simulink model "Testbench_for_Power_Circulating_TopologyA"  (R2023b)
settings: Solver=VariableStepAuto  StartTime=0.0  StopTime=4  RelTol=1e-3
InitFcn:
  | Initialization_for_Testbench;
values from neighbouring files (symbols this model uses):
  Cdc = 180e-6    (= 0.00018)    [CurrentLoop.m]    (also in Initialization_for_ESS_3P_2L_220kW.m; Initialization_for_Testbench.m)
  Fnom_Grid = 50    [CurrentLoop.m]    (also in Initialization_for_ESS_3P_2L_220kW.m; Initialization_for_Testbench.m)
  Gain_for_ActiveDamping = 1    [Initialization_for_Testbench.m]
  Inom = Pnom/sqrt(3)/Unom_Grid    [CurrentLoop.m]    (also in Initialization_for_ESS_3P_2L_220kW.m; Initialization_for_Testbench.m)
  Ki_Idq = Kp_Idq*2*pi*2    (= 40.2123859659)    [Initialization_for_ESS_3P_2L_220kW.m]    (also in Initialization_for_Testbench.m = 1.26330936334)
  Ki_Udc = Kp_Udc*2*pi*10    (= 6283.18530718)    [Initialization_for_Testbench.m]
  Kp_Idq = L_grid/3/Ts_Control*3    (= 3.2)    [Initialization_for_ESS_3P_2L_220kW.m]    (also in Initialization_for_Testbench.m = 2.0106192983)
  Kp_Udc = 100    [Initialization_for_Testbench.m]
  L_grid = 200e-6    (= 0.0002)    [Initialization_for_ESS_3P_2L_220kW.m]    (also in Initialization_for_Testbench.m)
  Pnom = 220e3    (= 220000)    [CurrentLoop.m]    (also in Initialization_for_ESS_3P_2L_220kW.m; Initialization_for_Testbench.m = 2500000)
  Ts_Control = 62.5e-6    (= 6.25e-05)    [CurrentLoop.m]    (also in Initialization_for_ESS_3P_2L_220kW.m; Initialization_for_Testbench.m = 0.0001)
  Ts_Power = 10e-7    (= 1e-06)    [Initialization_for_ESS_3P_2L_220kW.m]    (also in Initialization_for_Testbench.m)
  Udc_ref = 1500    [CurrentLoop.m]    (also in Initialization_for_ESS_3P_2L_220kW.m; Initialization_for_Testbench.m)
  Unom_Grid = 690    [CurrentLoop.m]    (also in Initialization_for_ESS_3P_2L_220kW.m; Initialization_for_Testbench.m)
  Unom_Phase = Unom_Grid/sqrt(3)    [CurrentLoop.m]    (also in Initialization_for_ESS_3P_2L_220kW.m; Initialization_for_Testbench.m)
libraries: LibraryForCodeGeneration x35, spsSeriesRLCBranchLib x3, spsThreePhaseVIMeasurementLib x3, spsTriangleGeneratorLib x2, spsThreePhaseSeriesRLCBranchLib x2, spsUniversalBridgeLib x2, eeProgrammableSignalGenerator x1, spsStairGeneratorLib x1, spsThreePhaseSourceLib x1, spsVoltageMeasurementLib x1, spspowerguiLib x1
settings Model: DataDictionary=VariablesDictionary_for_Testbench_TopologyA.sldd  Creator=ZZY  LastModifiedBy=ZZY

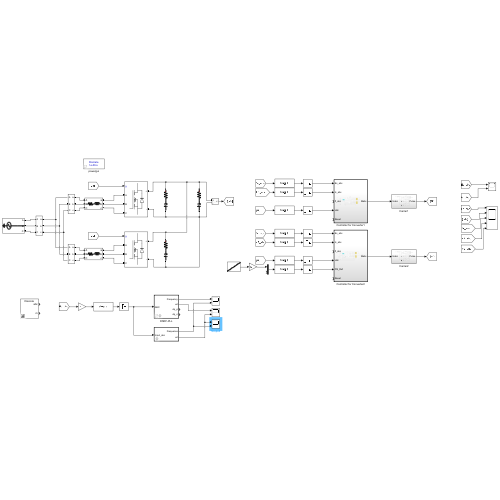
[thumbnail: Simulink's stored preview of the top-level diagram]
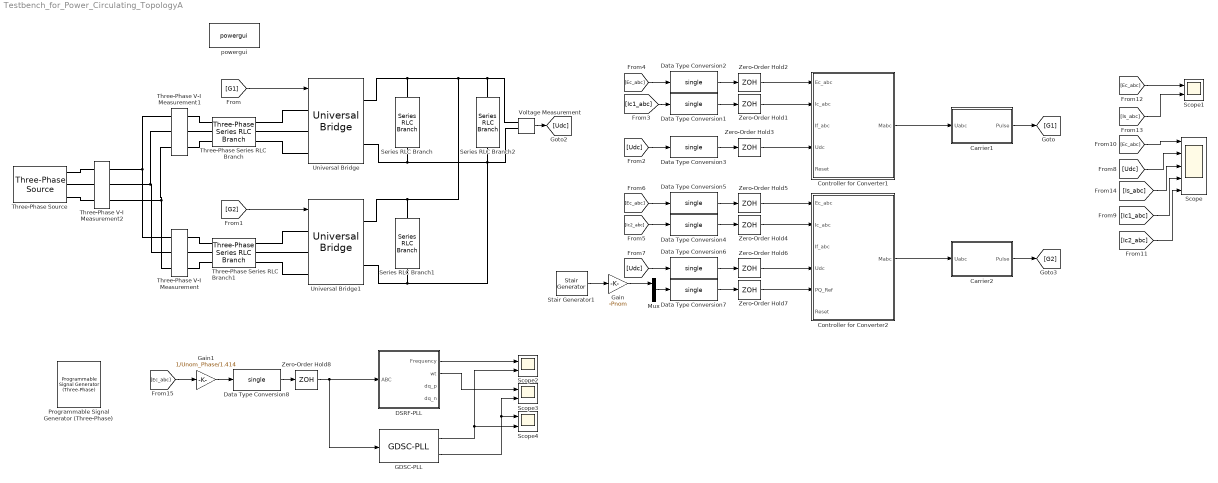
== system Testbench_for_Power_Circulating_TopologyA ==
  Carrier1 : Subsystem
  Carrier2 : Subsystem
  Controller for Converter1 : Subsystem  TreatAsAtomicUnit=on  SystemSampleTime=Ts_Control
  Controller for Converter2 : Subsystem  TreatAsAtomicUnit=on  SystemSampleTime=Ts_Control
  DSRF-PLL : Subsystem  AncestorBlock=LibraryForCodeGeneration/DSRF-PLL  TreatAsAtomicUnit=on  RTWFcnName=DSRF_PLL  mask{Ts=Ts_Control}
      mask prompts: Ts "Sampling Time:"
      settings: RTWFcnNameOpts=User specified
  Data Type Conversion{1..8} (8 alike) : DataTypeConversion  OutDataTypeStr=single  SaturateOnIntegerOverflow=off  RndMeth=Floor
  GDSC-PLL : LibraryForCodeGeneration/GDSC-PLL  Ts=Ts_Control  Fnom_Grid=50
  Gain : Gain  Gain=-Pnom
  Gain1 : Gain  Gain=1/Unom_Phase/1.414
  Mux : Mux  Inputs=2
  Programmable Signal Generator (Three-Phase) : eeProgrammableSignalGenerator/Programmable Signal Generator (Three-Phase)  LabelModeActiveChoice=Discrete  VariationAmplitude=Constant  Amp=0.8  Amp_RampRate=100  Amp_StepValue=100  Amp_ModulationMag=50  Amp_ModulationFreq=10  Amp_Tstart=0.1  Amp_Tstop=0.6  Amp_Table=[0 30 60 90]  Amp_Time=[0 0.3 0.6 0.9]  VariationFrequency=Constant  Freq=50  Freq_RampRate=100  Freq_StepValue=100  Freq_ModulationMag=50  Freq_ModulationFreq=10  Freq_Tstart=0.1  Freq_Tstop=0.6  Freq_Table=[0 30 60 90]  Freq_Time=[0 0.3 0.6 0.9]  VariationPhase=Constant  Phase=0  Phase_RampRate=100  Phase_StepValue=100  Phase_ModulationMag=50  Phase_ModulationFreq=10  Phase_Tstart=0.1  Phase_Tstop=0.6  Phase_Table=[0 30 60 90]  Phase_Time=[0 0.3 0.6 0.9]  Harmo_En1=on  Harmo_Seq1=Negative Sequence  Harmo_Ord1=2  Harmo_Mag1=0.4  Harmo_Phase1=180  Harmo_Tstart1=0.1  Harmo_Tstop1=0.6  Harmo_En2=on  Harmo_Seq2=Negative Sequence  Harmo_Ord2=3  Harmo_Mag2=0.4  Harmo_Phase2=180  Harmo_Tstart2=0.3  Harmo_Tstop2=1  Ts=Ts_Control
      settings: LibrarySourceBlock=|
      | ee_sl_lib/General Control/Programmable
      | Signal Generator (Three-Phase)
  Scope : Scope  NumInputPorts=5
  Scope{1..4} (4 alike) : Scope  NumInputPorts=2
  Series RLC Branch : spsSeriesRLCBranchLib/Series RLC Branch  LConnTagsString=__new0  RConnTagsString=__new0  BranchType=RC  Resistance=1e-6  Inductance=1e-3  SetiL0=off  InitialCurrent=0  Capacitance=Cdc  Setx0=on  InitialVoltage=Udc_ref  Measurements=Branch voltage
  Series RLC Branch1 : spsSeriesRLCBranchLib/Series RLC Branch  LConnTagsString=__new0  RConnTagsString=__new0  BranchType=RC  Resistance=1e-6  Inductance=1e-3  SetiL0=off  InitialCurrent=0  Capacitance=Cdc  Setx0=on  InitialVoltage=Udc_ref  Measurements=Branch voltage
  Series RLC Branch2 : spsSeriesRLCBranchLib/Series RLC Branch  LConnTagsString=__new0  RConnTagsString=__new0  BranchType=RC  Resistance=1e-6  Inductance=1e-3  SetiL0=off  InitialCurrent=0  Capacitance=Cdc*1000  Setx0=on  InitialVoltage=Udc_ref  Measurements=Branch voltage
  Stair Generator1 : spsStairGeneratorLib/Stair Generator  t=0:0.2:2  e=0:0.1:1  Ts=0
  Three-Phase Series RLC Branch : spsThreePhaseSeriesRLCBranchLib/Three-Phase Series RLC Branch  LConnTagsString=A|B|C  RConnTagsString=A|B|C  BranchType=RL  Resistance=1e-3  Inductance=L_grid*1  Capacitance=1e-6  Measurements=None
  Three-Phase Series RLC Branch1 : spsThreePhaseSeriesRLCBranchLib/Three-Phase Series RLC Branch  LConnTagsString=A|B|C  RConnTagsString=A|B|C  BranchType=RL  Resistance=1e-3  Inductance=L_grid*1  Capacitance=1e-6  Measurements=None
  Three-Phase V-I Measurement : spsThreePhaseVIMeasurementLib/Three-Phase V-I Measurement  VoltageMeasurement=no  SetLabelV=off  LabelV=Vabc  Vpu=off  VpuLL=off  CurrentMeasurement=yes  SetLabelI=on  LabelI=Ic2_abc  Ipu=off  Pbase=100e6  Vbase=500e3  OutputType=Complex  PhasorSimulation=off  PSBequivalent=0
  Three-Phase V-I Measurement1 : spsThreePhaseVIMeasurementLib/Three-Phase V-I Measurement  VoltageMeasurement=phase-to-phase  SetLabelV=on  LabelV=Ec_abc  Vpu=off  VpuLL=off  CurrentMeasurement=yes  SetLabelI=on  LabelI=Ic1_abc  Ipu=off  Pbase=100e6  Vbase=500e3  OutputType=Complex  PhasorSimulation=off  PSBequivalent=0
  Three-Phase V-I Measurement2 : spsThreePhaseVIMeasurementLib/Three-Phase V-I Measurement  VoltageMeasurement=no  SetLabelV=off  LabelV=Ec_abc  Vpu=off  VpuLL=off  CurrentMeasurement=yes  SetLabelI=on  LabelI=Is_abc  Ipu=off  Pbase=100e6  Vbase=500e3  OutputType=Complex  PhasorSimulation=off  PSBequivalent=0
  Three-Phase Source : spsThreePhaseSourceLib/Three-Phase Source  InternalConnection=Yg  VoltagePhases=off  Voltage=Unom_Grid  PhaseAngle=0  Voltage_phases=[25e3 25e3 25e3]/sqrt(3)  PhaseAngles_phases=[0 -120 +120]  Frequency=50  NonIdealSource=off  SpecifyImpedance=off  Resistance=0.08929  Inductance=2e-3  ShortCircuitLevel=100e6  BaseVoltage=Unom_Grid  XRratio=7  BusType=swing  Pref=10e3  Qref=0  Prefabc=[10e3, 10e3, 10e3]  Qrefabc=[0, 0, 0]  Qmin=-inf  Qmax=inf
  Universal Bridge : spsUniversalBridgeLib/Universal Bridge  Arms=3  SnubberResistance=1e5  SnubberCapacitance=inf  Device=MOSFET / Diodes  Ron=1e-3  Lon=0  ForwardVoltages="[  0  0  ]"  ForwardVoltage=0  GTOparameters=[ 10e-6 , 20e-6 ]  IGBTparameters=[ 1e-6 , 2e-6 ]  Measurements=None  Measurements_2=None  converterType=Rectifier
  Universal Bridge1 : spsUniversalBridgeLib/Universal Bridge  Arms=3  SnubberResistance=1e5  SnubberCapacitance=inf  Device=MOSFET / Diodes  Ron=1e-3  Lon=0  ForwardVoltages="[  0  0  ]"  ForwardVoltage=0  GTOparameters=[ 10e-6 , 20e-6 ]  IGBTparameters=[ 1e-6 , 2e-6 ]  Measurements=None  Measurements_2=None  converterType=Rectifier
  Voltage Measurement : spsVoltageMeasurementLib/Voltage Measurement  PhasorSimulation=off  OutputType=Complex  PSBequivalent=0
  Zero-Order Hold{1..8} (8 alike) : ZeroOrderHold  SampleTime=Ts_Control
  powergui : spspowerguiLib/powergui  Priority=1  SimulationMode=Discrete  SampleTime=Ts_Power  frequency=60  Iterations=50  frequencyindice=0  Pbase=100e6  ErrMax=1e-4  UnitsV=kV  UnitsW=MW  buscounter=0  FunctionMessages=off  echomessages=off  EnableUseOfTLC=off  CurrentSourceSwitches=off  DisableSnubberDevices=off  DisableRonSwitches=off  DisableVfSwitches=off  DisplayEquations=off  AutomaticDiscreteSolvers=off  SolverType=Tustin/Backward Euler (TBE)  Interpol=off  ExternalGateDelay=off  methode=off  Ts=100  x0status=blocks  SPID=on  SwTol=0  HookPort=off  NonlinearTolerance=1e-4  nMaxIteration=100  ContinueOnMaxIteration=off  RestoreLinks=warning  ResistiveCurrentMeasurement=off  Frange=[0:2:500]  Ylog=off  Xlog=on  ShowGrid=off  save=off  variable=ZData  structure=CHB_abc  ZoomFFT=off  StartTime=1.4  cycles=5  DisplayStyle=1  fundamental=50  FreqAxis=off  MaxFrequency=30000  frequencyindicesteady=1  RmsSteady=1  display=off
  wires:
  [G1] -> Universal Bridge/1
  [G2] -> Universal Bridge1/1
  Voltage Measurement/1 -> [Udc]
  Carrier1/1(Pulse) -> [G1]
  Carrier2/1(Pulse) -> [G2]
  Controller for Converter1/1(Mabc) -> Carrier1/1(Uabc)
  Controller for Converter2/1(Mabc) -> Carrier2/1(Uabc)
  Data Type Conversion3/1 -> Zero-Order Hold3/1
  [Udc] -> Data Type Conversion3/1
  Zero-Order Hold3/1 -> Controller for Converter1/4(Udc)
  [Ic1_abc] -> Data Type Conversion1/1
  Data Type Conversion1/1 -> Zero-Order Hold1/1
  Data Type Conversion2/1 -> Zero-Order Hold2/1
  [Ec_abc] -> Data Type Conversion2/1
  Zero-Order Hold2/1 -> Controller for Converter1/1(Ec_abc)
  Zero-Order Hold1/1 -> Controller for Converter1/2(Ic_abc)
  Data Type Conversion5/1 -> Zero-Order Hold5/1
  [Ic2_abc] -> Data Type Conversion4/1
  Data Type Conversion4/1 -> Zero-Order Hold4/1
  [Ec_abc] -> Data Type Conversion5/1
  Zero-Order Hold5/1 -> Controller for Converter2/1(Ec_abc)
  Zero-Order Hold4/1 -> Controller for Converter2/2(Ic_abc)
  Data Type Conversion6/1 -> Zero-Order Hold6/1
  [Udc] -> Data Type Conversion6/1
  Zero-Order Hold6/1 -> Controller for Converter2/4(Udc)
  [Udc] -> Scope/2
  [Ic1_abc] -> Scope/4
  [Ec_abc] -> Scope/1
  [Ic2_abc] -> Scope/5
  Mux/1 -> Data Type Conversion7/1
  Data Type Conversion7/1 -> Zero-Order Hold7/1
  Zero-Order Hold7/1 -> Controller for Converter2/5(PQ_Ref)
  Gain/1 -> Mux/1
  Stair Generator1/1 -> Gain/1
  [Ec_abc] -> Scope1/1
  [Is_abc] -> Scope1/2
  [Is_abc] -> Scope/3
  [Ec_abc] -> Gain1/1
  Data Type Conversion8/1 -> Zero-Order Hold8/1
  DSRF-PLL/1(Frequency) -> Scope2/1
  GDSC-PLL/1 -> Scope4/2, Scope2/2
  DSRF-PLL/2(wt) -> Scope3/1
  GDSC-PLL/2 -> Scope4/1, Scope3/2
  Zero-Order Hold8/1 -> GDSC-PLL/1, DSRF-PLL/1(ABC)
  Gain1/1 -> Data Type Conversion8/1
  connections:
  Series RLC Branch1/LConn1 -- Series RLC Branch2/LConn1 -- Voltage Measurement/LConn1 -- Universal Bridge/RConn1 -- Series RLC Branch/LConn1 -- Universal Bridge1/RConn1
  Series RLC Branch1/RConn1 -- Universal Bridge/RConn2 -- Series RLC Branch/RConn1 -- Voltage Measurement/LConn2 -- Series RLC Branch2/RConn1 -- Universal Bridge1/RConn2
  Three-Phase Series RLC Branch/RConn2 -- Universal Bridge/LConn2
  Three-Phase Series RLC Branch/RConn1 -- Universal Bridge/LConn1
  Three-Phase Series RLC Branch/RConn3 -- Universal Bridge/LConn3
  Three-Phase V-I Measurement1/LConn3 -- Three-Phase V-I Measurement2/RConn3 -- Three-Phase V-I Measurement/LConn3
  Three-Phase V-I Measurement1/LConn2 -- Three-Phase V-I Measurement2/RConn2 -- Three-Phase V-I Measurement/LConn2
  Three-Phase V-I Measurement1/LConn1 -- Three-Phase V-I Measurement2/RConn1 -- Three-Phase V-I Measurement/LConn1
  Three-Phase V-I Measurement1/RConn2 -- Three-Phase Series RLC Branch/LConn2
  Three-Phase V-I Measurement1/RConn1 -- Three-Phase Series RLC Branch/LConn1
  Three-Phase V-I Measurement1/RConn3 -- Three-Phase Series RLC Branch/LConn3
  Three-Phase Series RLC Branch1/LConn2 -- Three-Phase V-I Measurement/RConn2
  Three-Phase V-I Measurement/RConn1 -- Three-Phase Series RLC Branch1/LConn1
  Three-Phase V-I Measurement/RConn3 -- Three-Phase Series RLC Branch1/LConn3
  Three-Phase Series RLC Branch1/RConn2 -- Universal Bridge1/LConn2
  Three-Phase Series RLC Branch1/RConn1 -- Universal Bridge1/LConn1
  Three-Phase Series RLC Branch1/RConn3 -- Universal Bridge1/LConn3
  Three-Phase V-I Measurement2/LConn2 -- Three-Phase Source/RConn2
  Three-Phase Source/RConn1 -- Three-Phase V-I Measurement2/LConn1
  Three-Phase Source/RConn3 -- Three-Phase V-I Measurement2/LConn3

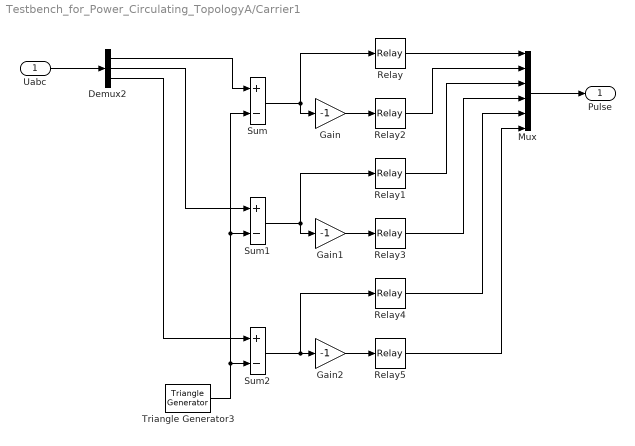
== system Testbench_for_Power_Circulating_TopologyA/Carrier1 ==
  Uabc : Inport
  Demux2 : Demux  Outputs=3
  Gain : Gain  Gain=-1
  Gain1 : Gain  Gain=-1
  Gain2 : Gain  Gain=-1
  Mux : Mux  Inputs=6
  Relay{,1..5} (6 alike) : Relay  OffSwitchValue=-eps
  Sum : Sum  Inputs=+-
  Sum1 : Sum  Inputs=+-
  Sum2 : Sum  Inputs=+-
  Triangle Generator3 : spsTriangleGeneratorLib/Triangle Generator  Freq=Fsw  Phase=180  Ts=1e-6
  Pulse : Outport
  wires:
  Mux/1 -> Pulse/1
  Gain/1 -> Relay2/1
  Sum/1 -> Relay/1, Gain/1
  Uabc/1 -> Demux2/1
  Demux2/1 -> Sum/1
  Relay/1 -> Mux/1
  Relay2/1 -> Mux/2
  Relay1/1 -> Mux/3
  Relay3/1 -> Mux/4
  Gain1/1 -> Relay3/1
  Demux2/2 -> Sum1/1
  Sum1/1 -> Relay1/1, Gain1/1
  Relay5/1 -> Mux/6
  Demux2/3 -> Sum2/1
  Gain2/1 -> Relay5/1
  Sum2/1 -> Relay4/1, Gain2/1
  Relay4/1 -> Mux/5
  Triangle Generator3/1 -> Sum/2, Sum1/2, Sum2/2

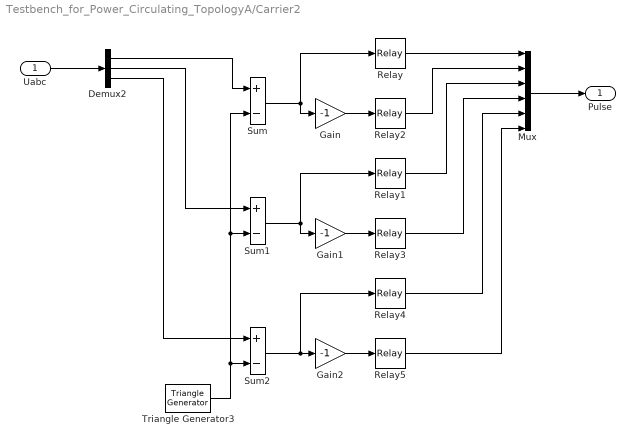
== system Testbench_for_Power_Circulating_TopologyA/Carrier2 ==
  Uabc : Inport
  Demux2 : Demux  Outputs=3
  Gain : Gain  Gain=-1
  Gain1 : Gain  Gain=-1
  Gain2 : Gain  Gain=-1
  Mux : Mux  Inputs=6
  Relay{,1..5} (6 alike) : Relay  OffSwitchValue=-eps
  Sum : Sum  Inputs=+-
  Sum1 : Sum  Inputs=+-
  Sum2 : Sum  Inputs=+-
  Triangle Generator3 : spsTriangleGeneratorLib/Triangle Generator  Freq=Fsw  Phase=180  Ts=1e-6
  Pulse : Outport
  wires:
  Triangle Generator3/1 -> Sum2/2, Sum1/2, Sum/2
  Relay4/1 -> Mux/5
  Sum2/1 -> Gain2/1, Relay4/1
  Gain2/1 -> Relay5/1
  Demux2/3 -> Sum2/1
  Relay5/1 -> Mux/6
  Sum1/1 -> Gain1/1, Relay1/1
  Demux2/2 -> Sum1/1
  Gain1/1 -> Relay3/1
  Relay3/1 -> Mux/4
  Relay1/1 -> Mux/3
  Relay2/1 -> Mux/2
  Relay/1 -> Mux/1
  Demux2/1 -> Sum/1
  Uabc/1 -> Demux2/1
  Sum/1 -> Gain/1, Relay/1
  Gain/1 -> Relay2/1
  Mux/1 -> Pulse/1

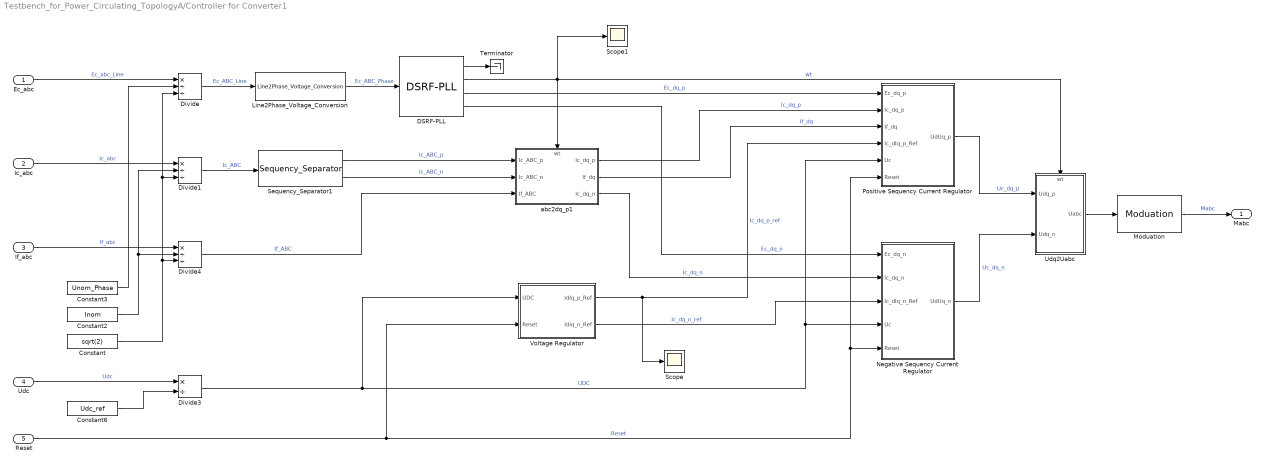
== system Testbench_for_Power_Circulating_TopologyA/Controller for Converter1 ==
  Ec_abc : Inport  OutDataTypeStr=single
  Ic_abc : Inport  Port=2  OutDataTypeStr=single
  If_abc : Inport  Port=3  OutDataTypeStr=single
  Udc : Inport  Port=4  OutDataTypeStr=single
  Reset : Inport  Port=5  OutDataTypeStr=boolean
  Constant : Constant  Value=sqrt(2)  OutDataTypeStr=Inherit: Inherit via back propagation  SampleTime=-1
  Constant2 : Constant  Value=Inom  OutDataTypeStr=Inherit: Inherit via back propagation  SampleTime=-1
  Constant3 : Constant  Value=Unom_Phase  OutDataTypeStr=Inherit: Inherit via back propagation  SampleTime=-1
  Constant6 : Constant  Value=Udc_ref  OutDataTypeStr=Inherit: Inherit via back propagation  SampleTime=-1
  DSRF-PLL : LibraryForCodeGeneration/DSRF-PLL  Ts=Ts_Control
  Divide : Product  Inputs=*//  OutDataTypeStr=single
  Divide1 : Product  Inputs=*//  OutDataTypeStr=single
  Divide3 : Product  Inputs=*/  OutDataTypeStr=single
  Divide4 : Product  Inputs=*//  OutDataTypeStr=single
  Line2Phase_Voltage_Conversion : LibraryForCodeGeneration/Line2Phase_Voltage_Conversion  SystemSampleTime=-1  VariantActivationTime=update diagram  AllowFlexibleInterface=on  Latency=0  AutoFrameSizeCalculation=off
  Moduation : LibraryForCodeGeneration/Moduation  Modulation=SPWM
  Negative Sequency Current Regulator : Subsystem
  Positive Sequency Current Regulator : Subsystem
  Scope : Scope
  Scope1 : Scope
  Sequency_Separator1 : LibraryForCodeGeneration/Sequency_Separator  SystemSampleTime=-1  VariantActivationTime=update diagram  AllowFlexibleInterface=on  Latency=0  AutoFrameSizeCalculation=off
  Terminator : Terminator
  Udq2Uabc : Subsystem
      settings: PortSchema="{\"entries\":[{\"content\":{\"sides\":[{\"content\":{\"connectorIds\":[\"In1\",\"In2\"]},\"type\":\"ConnectorPlacement.EquallySpacedRectSide\",\"uuid\":\"009786f4-728c-4160-b9bf-eaf0b5a05101\"},{\"content\":{\"connectorIds\":[\"Out1\"],\"side\":\"RIGHT\"},\"type\":\"ConnectorPlacement.EquallySpacedRectSide\",\"uuid\":\"2a94367a-5c57-4632-9573-ab089470159a\"},{\"content\":{\"connectorIds\":[\"In3\"],\"side\":\"TOP\"},\"type\":\"ConnectorPlacement.EquallySpacedRectSide\",\"uuid\":\"6906365b-3187-4c4b-97cf-c9dec4c5ef7c\"}]},\"type\":\"ConnectorPlacement.EquallySpacedConnector\",\"uuid\":\"96ca8566-a266-405c-817a-b47b433d51ed\"}],\"packageUris\":[\"http://schema.mathworks.com/mf0/Connector/R2020b\"],\"version\":\"1.0\"}"
  Voltage Regulator : Subsystem
  abc2dq_p1 : Subsystem
      settings: PortSchema="{\"entries\":[{\"content\":{\"sides\":[{\"content\":{\"connectorIds\":[\"In1\",\"In2\",\"In3\"]},\"type\":\"ConnectorPlacement.EquallySpacedRectSide\",\"uuid\":\"702c7fae-dbbb-427d-af19-afd468018ae6\"},{\"content\":{\"connectorIds\":[\"Out1\",\"Out2\",\"Out3\"],\"side\":\"RIGHT\"},\"type\":\"ConnectorPlacement.EquallySpacedRectSide\",\"uuid\":\"d2ca5462-a446-46d8-bb73-1a455ffa959f\"},{\"content\":{\"connectorIds\":[\"In4\"],\"side\":\"TOP\"},\"type\":\"ConnectorPlacement.EquallySpacedRectSide\",\"uuid\":\"50bc6c44-424f-4342-960e-11540364fe97\"}]},\"type\":\"ConnectorPlacement.EquallySpacedConnector\",\"uuid\":\"f58cf64d-fe35-43f1-a031-7ee625a8bb1e\"}],\"packageUris\":[\"http://schema.mathworks.com/mf0/Connector/R2020b\"],\"version\":\"1.0\"}"
  Mabc : Outport  OutDataTypeStr=single
  wires:
  Divide3/1 -> Voltage Regulator/1(UDC), Positive Sequency Current Regulator/5(Uc), Negative Sequency Current Regulator/4(Uc)  "UDC"
  Positive Sequency Current Regulator/1(UdUq_p) -> Udq2Uabc/1(Udq_p)  "Uc_dq_p"
  Divide4/1 -> abc2dq_p1/3(If_ABC)  "If_ABC"
  Sequency_Separator1/1 -> abc2dq_p1/1("Ic_ABC_p ")  "Ic_ABC_p"
  If_abc/1 -> Divide4/1  "If_abc"
  DSRF-PLL/4 -> Negative Sequency Current Regulator/1(Ec_dq_n)  "Ec_dq_n"
  DSRF-PLL/2 -> Scope1/1, Udq2Uabc/3(wt), abc2dq_p1/4(wt)  "wt"
  abc2dq_p1/1(Ic_dq_p) -> Positive Sequency Current Regulator/2(Ic_dq_p)  "Ic_dq_p"
  Reset/1 -> Voltage Regulator/2(Reset), Positive Sequency Current Regulator/6(Reset), Negative Sequency Current Regulator/5(Reset)  "Reset"
  Moduation/1 -> Mabc/1  "Mabc"
  DSRF-PLL/1 -> Terminator/1
  abc2dq_p1/2(If_dq) -> Positive Sequency Current Regulator/3(If_dq)  "If_dq"
  Constant2/1 -> Divide4/2, Divide1/2
  Constant/1 -> Divide4/3, Divide1/3, Divide/3
  Voltage Regulator/1(IdIq_p_Ref) -> Scope/1, Positive Sequency Current Regulator/4(Ic_dIq_p_Ref)  "Ic_dq_p_ref"
  Udq2Uabc/1(Uabc) -> Moduation/1
  Voltage Regulator/2(IdIq_n_Ref) -> Negative Sequency Current Regulator/3(Ic_dIq_n_Ref)  "Ic_dq_n_ref"
  Constant3/1 -> Divide/2
  Constant6/1 -> Divide3/2
  DSRF-PLL/3 -> Positive Sequency Current Regulator/1(Ec_dq_p)  "Ec_dq_p"
  Divide1/1 -> Sequency_Separator1/1  "Ic_ABC"
  Udc/1 -> Divide3/1  "Udc"
  Sequency_Separator1/2 -> abc2dq_p1/2("Ic_ABC_n ")  "Ic_ABC_n"
  Ic_abc/1 -> Divide1/1  "Ic_abc"
  Ec_abc/1 -> Divide/1  "Ec_abc_Line"
  Divide/1 -> Line2Phase_Voltage_Conversion/1  "Ec_ABC_Line"
  Line2Phase_Voltage_Conversion/1 -> DSRF-PLL/1  "Ec_ABC_Phase"
  abc2dq_p1/3(Ic_dq_n) -> Negative Sequency Current Regulator/2(Ic_dq_n)  "Ic_dq_n"
  Negative Sequency Current Regulator/1(UdUq_n) -> Udq2Uabc/2(Udq_n)  "Uc_dq_n"

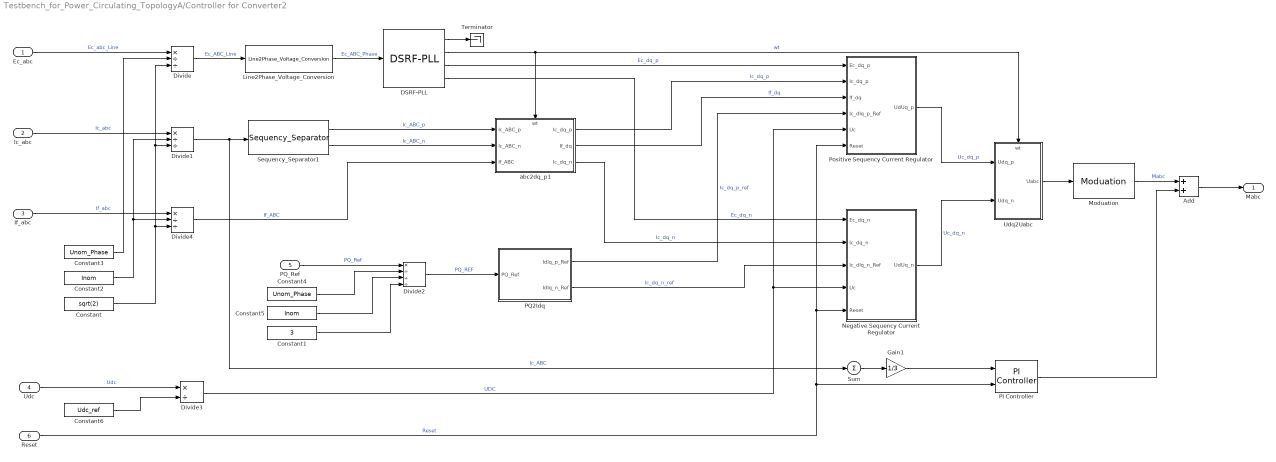
== system Testbench_for_Power_Circulating_TopologyA/Controller for Converter2 ==
  Ec_abc : Inport  OutDataTypeStr=single
  Ic_abc : Inport  Port=2  OutDataTypeStr=single
  If_abc : Inport  Port=3  OutDataTypeStr=single
  Udc : Inport  Port=4  OutDataTypeStr=single
  PQ_Ref : Inport  Port=5  OutDataTypeStr=single
  Reset : Inport  Port=6  OutDataTypeStr=boolean
  Add : Sum
  Constant : Constant  Value=sqrt(2)  OutDataTypeStr=Inherit: Inherit via back propagation  SampleTime=-1
  Constant1 : Constant  Value=3  OutDataTypeStr=Inherit: Inherit via back propagation  SampleTime=-1
  Constant2 : Constant  Value=Inom  OutDataTypeStr=Inherit: Inherit via back propagation  SampleTime=-1
  Constant3 : Constant  Value=Unom_Phase  OutDataTypeStr=Inherit: Inherit via back propagation  SampleTime=-1
  Constant4 : Constant  Value=Unom_Phase  OutDataTypeStr=Inherit: Inherit via back propagation  SampleTime=-1
  Constant5 : Constant  Value=Inom  OutDataTypeStr=Inherit: Inherit via back propagation  SampleTime=-1
  Constant6 : Constant  Value=Udc_ref  OutDataTypeStr=Inherit: Inherit via back propagation  SampleTime=-1
  DSRF-PLL : LibraryForCodeGeneration/DSRF-PLL  Ts=Ts_Control
  Divide : Product  Inputs=*//  OutDataTypeStr=single
  Divide1 : Product  Inputs=*//  OutDataTypeStr=single
  Divide2 : Product  Inputs=*///  OutDataTypeStr=single
  Divide3 : Product  Inputs=*/  OutDataTypeStr=single
  Divide4 : Product  Inputs=*//  OutDataTypeStr=single
  Gain1 : Gain  Gain=1/3
  Line2Phase_Voltage_Conversion : LibraryForCodeGeneration/Line2Phase_Voltage_Conversion  SystemSampleTime=-1  VariantActivationTime=update diagram  AllowFlexibleInterface=on  Latency=0  AutoFrameSizeCalculation=off
  Moduation : LibraryForCodeGeneration/Moduation  Modulation=SPWM
  Negative Sequency Current Regulator : Subsystem
  PI Controller : LibraryForCodeGeneration/PI Controller  Kp=1  Ki=0.001  Ts=Ts_Control  Max=2  Min=-2
  PQ2Idq : Subsystem
  Positive Sequency Current Regulator : Subsystem
  Sequency_Separator1 : LibraryForCodeGeneration/Sequency_Separator  SystemSampleTime=-1  VariantActivationTime=update diagram  AllowFlexibleInterface=on  Latency=0  AutoFrameSizeCalculation=off
  Sum : Sum  Inputs=+
  Terminator : Terminator
  Udq2Uabc : Subsystem
      settings: PortSchema="{\"entries\":[{\"content\":{\"sides\":[{\"content\":{\"connectorIds\":[\"In1\",\"In2\"]},\"type\":\"ConnectorPlacement.EquallySpacedRectSide\",\"uuid\":\"009786f4-728c-4160-b9bf-eaf0b5a05101\"},{\"content\":{\"connectorIds\":[\"Out1\"],\"side\":\"RIGHT\"},\"type\":\"ConnectorPlacement.EquallySpacedRectSide\",\"uuid\":\"2a94367a-5c57-4632-9573-ab089470159a\"},{\"content\":{\"connectorIds\":[\"In3\"],\"side\":\"TOP\"},\"type\":\"ConnectorPlacement.EquallySpacedRectSide\",\"uuid\":\"6906365b-3187-4c4b-97cf-c9dec4c5ef7c\"}]},\"type\":\"ConnectorPlacement.EquallySpacedConnector\",\"uuid\":\"96ca8566-a266-405c-817a-b47b433d51ed\"}],\"packageUris\":[\"http://schema.mathworks.com/mf0/Connector/R2020b\"],\"version\":\"1.0\"}"
  abc2dq_p1 : Subsystem
      settings: PortSchema="{\"entries\":[{\"content\":{\"sides\":[{\"content\":{\"connectorIds\":[\"In1\",\"In2\",\"In3\"]},\"type\":\"ConnectorPlacement.EquallySpacedRectSide\",\"uuid\":\"702c7fae-dbbb-427d-af19-afd468018ae6\"},{\"content\":{\"connectorIds\":[\"Out1\",\"Out2\",\"Out3\"],\"side\":\"RIGHT\"},\"type\":\"ConnectorPlacement.EquallySpacedRectSide\",\"uuid\":\"d2ca5462-a446-46d8-bb73-1a455ffa959f\"},{\"content\":{\"connectorIds\":[\"In4\"],\"side\":\"TOP\"},\"type\":\"ConnectorPlacement.EquallySpacedRectSide\",\"uuid\":\"50bc6c44-424f-4342-960e-11540364fe97\"}]},\"type\":\"ConnectorPlacement.EquallySpacedConnector\",\"uuid\":\"f58cf64d-fe35-43f1-a031-7ee625a8bb1e\"}],\"packageUris\":[\"http://schema.mathworks.com/mf0/Connector/R2020b\"],\"version\":\"1.0\"}"
  Mabc : Outport  OutDataTypeStr=single
  wires:
  Negative Sequency Current Regulator/1(UdUq_n) -> Udq2Uabc/2(Udq_n)  "Uc_dq_n"
  abc2dq_p1/3(Ic_dq_n) -> Negative Sequency Current Regulator/2(Ic_dq_n)  "Ic_dq_n"
  Line2Phase_Voltage_Conversion/1 -> DSRF-PLL/1  "Ec_ABC_Phase"
  Divide/1 -> Line2Phase_Voltage_Conversion/1  "Ec_ABC_Line"
  Ec_abc/1 -> Divide/1  "Ec_abc_Line"
  Ic_abc/1 -> Divide1/1  "Ic_abc"
  Sequency_Separator1/2 -> abc2dq_p1/2("Ic_ABC_n ")  "Ic_ABC_n"
  Udc/1 -> Divide3/1  "Udc"
  Divide1/1 -> Sum/1, Sequency_Separator1/1  "Ic_ABC"
  DSRF-PLL/3 -> Positive Sequency Current Regulator/1(Ec_dq_p)  "Ec_dq_p"
  Constant6/1 -> Divide3/2
  Constant3/1 -> Divide/2
  PQ2Idq/2(IdIq_n_Ref) -> Negative Sequency Current Regulator/3(Ic_dIq_n_Ref)  "Ic_dq_n_ref"
  Udq2Uabc/1(Uabc) -> Moduation/1
  PQ2Idq/1(IdIq_p_Ref) -> Positive Sequency Current Regulator/4(Ic_dIq_p_Ref)  "Ic_dq_p_ref"
  Constant/1 -> Divide/3, Divide1/3, Divide4/3
  Constant2/1 -> Divide1/2, Divide4/2
  abc2dq_p1/2(If_dq) -> Positive Sequency Current Regulator/3(If_dq)  "If_dq"
  DSRF-PLL/1 -> Terminator/1
  Constant5/1 -> Divide2/3
  Moduation/1 -> Add/1  "Mabc"
  Reset/1 -> PI Controller/2, Negative Sequency Current Regulator/5(Reset), Positive Sequency Current Regulator/6(Reset)  "Reset"
  abc2dq_p1/1(Ic_dq_p) -> Positive Sequency Current Regulator/2(Ic_dq_p)  "Ic_dq_p"
  DSRF-PLL/2 -> abc2dq_p1/4(wt), Udq2Uabc/3(wt)  "wt"
  DSRF-PLL/4 -> Negative Sequency Current Regulator/1(Ec_dq_n)  "Ec_dq_n"
  If_abc/1 -> Divide4/1  "If_abc"
  Constant4/1 -> Divide2/2
  Sequency_Separator1/1 -> abc2dq_p1/1("Ic_ABC_p ")  "Ic_ABC_p"
  Divide4/1 -> abc2dq_p1/3(If_ABC)  "If_ABC"
  Constant1/1 -> Divide2/4
  Positive Sequency Current Regulator/1(UdUq_p) -> Udq2Uabc/1(Udq_p)  "Uc_dq_p"
  PQ_Ref/1 -> Divide2/1  "PQ_Ref"
  Divide2/1 -> PQ2Idq/1(PQ_Ref)  "PQ_REF"
  Divide3/1 -> Negative Sequency Current Regulator/4(Uc), Positive Sequency Current Regulator/5(Uc)  "UDC"
  Gain1/1 -> PI Controller/1
  Sum/1 -> Gain1/1
  Add/1 -> Mabc/1
  PI Controller/1 -> Add/2

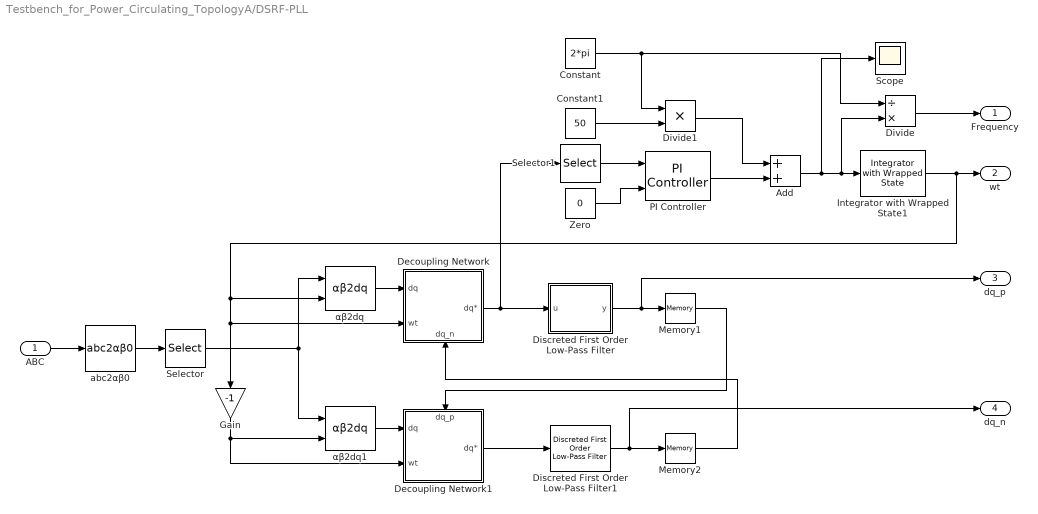
== system Testbench_for_Power_Circulating_TopologyA/DSRF-PLL ==
  ABC : Inport
  Add : Sum
  Constant : Constant  Value=2*pi  OutDataTypeStr=single  SampleTime=-1
  Constant1 : Constant  Value=50  OutDataTypeStr=Inherit: Inherit via back propagation  SampleTime=-1
  Decoupling Network : Subsystem
      settings: PortSchema="{\"entries\":[{\"content\":{\"sides\":[{\"content\":{\"connectorIds\":[\"In1\",\"In2\"]},\"type\":\"ConnectorPlacement.EquallySpacedRectSide\",\"uuid\":\"616b24e1-56e6-4614-ba2f-bd62e326c103\"},{\"content\":{\"connectorIds\":[\"Out1\"],\"side\":\"RIGHT\"},\"type\":\"ConnectorPlacement.EquallySpacedRectSide\",\"uuid\":\"d002ccc8-a8e9-4a33-b4ba-37ade36bc88e\"},{\"content\":{\"side\":\"TOP\"},\"type\":\"ConnectorPlacement.EquallySpacedRectSide\",\"uuid\":\"22e49a5d-b55b-4fa7-ad37-ecfc3ef17bd3\"},{\"content\":{\"connectorIds\":[\"In3\"],\"side\":\"BOTTOM\"},\"type\":\"ConnectorPlacement.EquallySpacedRectSide\",\"uuid\":\"7e8d98ba-e876-4857-9b05-7c0be2a1c9ed\"}]},\"type\":\"ConnectorPlacement.EquallySpacedConnector\",\"uuid\":\"40cd40bf-343a-4150-bffd-169ac481916a\"}],\"packageUris\":[\"http://schema.mathworks.com/mf0/Connector/R2020b\"],\"version\":\"1.0\"}"
  Decoupling Network1 : Subsystem
      settings: PortSchema="{\"entries\":[{\"content\":{\"sides\":[{\"content\":{\"connectorIds\":[\"In1\",\"In2\"]},\"type\":\"ConnectorPlacement.EquallySpacedRectSide\",\"uuid\":\"616b24e1-56e6-4614-ba2f-bd62e326c103\"},{\"content\":{\"connectorIds\":[\"Out1\"],\"side\":\"RIGHT\"},\"type\":\"ConnectorPlacement.EquallySpacedRectSide\",\"uuid\":\"d002ccc8-a8e9-4a33-b4ba-37ade36bc88e\"},{\"content\":{\"connectorIds\":[\"In3\"],\"side\":\"TOP\"},\"type\":\"ConnectorPlacement.EquallySpacedRectSide\",\"uuid\":\"22e49a5d-b55b-4fa7-ad37-ecfc3ef17bd3\"}]},\"type\":\"ConnectorPlacement.EquallySpacedConnector\",\"uuid\":\"40cd40bf-343a-4150-bffd-169ac481916a\"}],\"packageUris\":[\"http://schema.mathworks.com/mf0/Connector/R2020b\"],\"version\":\"1.0\"}"
  Discreted First Order Low-Pass Filter : Subsystem  TreatAsAtomicUnit=on  mask{Wc=2*pi*50*0.707, Ts=Ts}
      mask prompts: Wc "Cut-off Frequency (rad):"; Ts "Sample time (-1 for inherited):"
  Discreted First Order Low-Pass Filter1 : LibraryForCodeGeneration/DSRF-PLL/Discreted First Order Low-Pass Filter  Wc=2*pi*50*0.707  Ts=Ts
  Divide : Product  Inputs=/*  OutDataTypeStr=Inherit: Inherit via back propagation
  Divide1 : Product  Inputs=**  OutDataTypeStr=Inherit: Inherit via back propagation
  Gain : Gain  Gain=-1
  Integrator with Wrapped State1 : LibraryForCodeGeneration/Integrator with Wrapped State  VariantControl=Discrete  WrappedStateUpperValue=2*pi  WrappedStateLowerValue=0  Ts=Ts
  Memory1 : Memory  InheritSampleTime=on
  Memory2 : Memory  InheritSampleTime=on
  PI Controller : LibraryForCodeGeneration/PI Controller  Kp=222  Ki=222*2*pi*17.7  Ts=Ts  Max=2*pi*100  Min=-2*pi*100
  Scope : Scope
  Selector : Selector  InputPortWidth=3  IndexOptions=Index vector (dialog)  Indices=[1 2]  OutputSizes=1
  Selector1 : Selector  InputPortWidth=2  IndexOptions=Index vector (dialog)  Indices=[2]  OutputSizes=1
  Zero : Constant  Value=0  OutDataTypeStr=boolean  SampleTime=-1
  abc2αβ0 : LibraryForCodeGeneration/abc2αβ0  SystemSampleTime=-1  VariantActivationTime=update diagram  AllowFlexibleInterface=on  Latency=0  AutoFrameSizeCalculation=off
  αβ2dq : LibraryForCodeGeneration/αβ2dq  SystemSampleTime=-1  VariantActivationTime=update diagram  AllowFlexibleInterface=on  Latency=0  AutoFrameSizeCalculation=off
  αβ2dq1 : LibraryForCodeGeneration/αβ2dq  SystemSampleTime=-1  VariantActivationTime=update diagram  AllowFlexibleInterface=on  Latency=0  AutoFrameSizeCalculation=off
  Frequency : Outport
  wt : Outport  Port=2
  dq_p : Outport  Port=3
  dq_n : Outport  Port=4
  wires:
  Discreted First Order Low-Pass Filter1/1 -> Memory2/1, dq_n/1
  Memory2/1 -> Decoupling Network/3(dq_n)
  Memory1/1 -> Decoupling Network1/3(dq_p)
  Zero/1 -> PI Controller/2
  Divide1/1 -> Add/1
  Constant1/1 -> Divide1/2
  PI Controller/1 -> Add/2
  Integrator with Wrapped State1/1 -> αβ2dq/2, Gain/1, Decoupling Network/2(wt), wt/1
  Discreted First Order Low-Pass Filter/1(y) -> Memory1/1, dq_p/1
  Divide/1 -> Frequency/1
  αβ2dq/1 -> Decoupling Network/1(dq)
  Selector1/1 -> PI Controller/1
  αβ2dq1/1 -> Decoupling Network1/1(dq)
  Decoupling Network1/1(dq*) -> Discreted First Order Low-Pass Filter1/1
  Constant/1 -> Divide1/1, Divide/1
  Gain/1 -> αβ2dq1/2, Decoupling Network1/2(wt)
  abc2αβ0/1 -> Selector/1
  ABC/1 -> abc2αβ0/1
  Add/1 -> Scope/1, Divide/2, Integrator with Wrapped State1/1
  Selector/1 -> αβ2dq/1, αβ2dq1/1
  Decoupling Network/1(dq*) -> Selector1/1, Discreted First Order Low-Pass Filter/1(u)

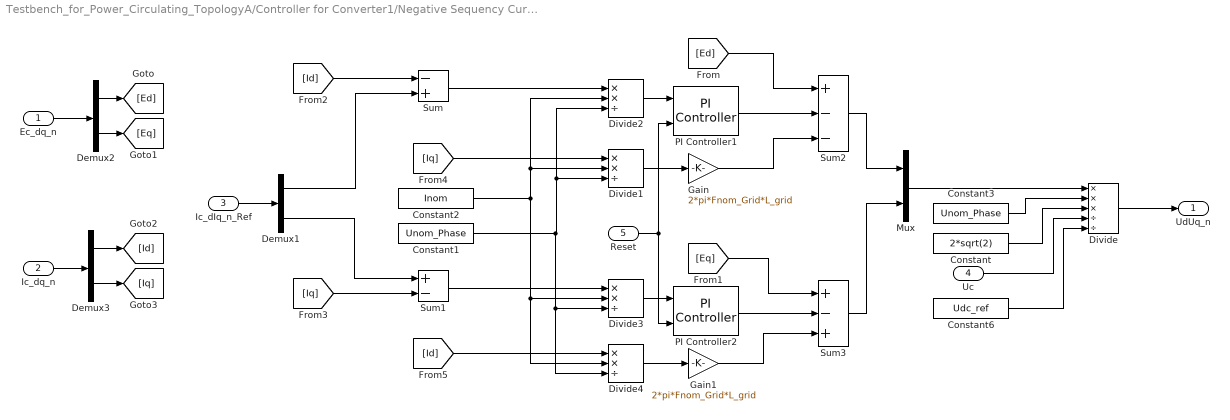
== system Testbench_for_Power_Circulating_TopologyA/Controller for Converter1/Negative Sequency Current Regulator ==
  Ec_dq_n : Inport
  Ic_dq_n : Inport  Port=2
  Ic_dIq_n_Ref : Inport  Port=3
  Uc : Inport  Port=4
  Reset : Inport  Port=5  OutDataTypeStr=boolean
  Constant : Constant  Value=2*sqrt(2)  OutDataTypeStr=Inherit: Inherit via back propagation  SampleTime=-1
  Constant1 : Constant  Value=Unom_Phase  OutDataTypeStr=Inherit: Inherit via back propagation  SampleTime=-1
  Constant2 : Constant  Value=Inom  OutDataTypeStr=Inherit: Inherit via back propagation  SampleTime=-1
  Constant3 : Constant  Value=Unom_Phase  OutDataTypeStr=Inherit: Inherit via back propagation  SampleTime=-1
  Constant6 : Constant  Value=Udc_ref  OutDataTypeStr=Inherit: Inherit via back propagation  SampleTime=-1
  Demux1 : Demux  Outputs=2
  Demux2 : Demux  Outputs=2
  Demux3 : Demux  Outputs=2
  Divide : Product  Inputs=***//  OutDataTypeStr=single
  Divide{1..4} (4 alike) : Product  Inputs=**/  OutDataTypeStr=single
  Gain : Gain  Gain=2*pi*Fnom_Grid*L_grid  ParamDataTypeStr=Inherit: Same as input
  Gain1 : Gain  Gain=2*pi*Fnom_Grid*L_grid  ParamDataTypeStr=Inherit: Same as input
  Mux : Mux  Inputs=2
  PI Controller1 : LibraryForCodeGeneration/PI Controller  Kp=Kp_Idq  Ki=Ki_Idq  Ts=Ts_Control  Max=2  Min=-2
  PI Controller2 : LibraryForCodeGeneration/PI Controller  Kp=Kp_Idq  Ki=Ki_Idq  Ts=Ts_Control  Max=2  Min=-2
  Sum : Sum  Inputs=-+  InputSameDT=on  SaturateOnIntegerOverflow=on  OutDataTypeStr=Inherit: Same as first input
  Sum1 : Sum  Inputs=+-  InputSameDT=on  SaturateOnIntegerOverflow=on  OutDataTypeStr=Inherit: Same as first input
  Sum2 : Sum  Inputs=+--  InputSameDT=on  SaturateOnIntegerOverflow=on  OutDataTypeStr=Inherit: Same as first input
  Sum3 : Sum  Inputs=+-+  InputSameDT=on  SaturateOnIntegerOverflow=on  OutDataTypeStr=Inherit: Same as first input
  UdUq_n : Outport
  wires:
  [Id] -> Divide4/1
  [Iq] -> Divide1/1
  [Iq] -> Sum1/2
  [Id] -> Sum/1
  Ic_dq_n/1 -> Demux3/1
  Demux3/1 -> [Id]
  Demux3/2 -> [Iq]
  Demux1/2 -> Sum1/1
  Demux1/1 -> Sum/2
  [Eq] -> Sum3/1
  [Ed] -> Sum2/1
  Demux2/2 -> [Eq]
  Demux2/1 -> [Ed]
  Divide3/1 -> PI Controller2/1
  Sum/1 -> Divide2/1
  Mux/1 -> Divide/1
  Divide/1 -> UdUq_n/1
  Gain1/1 -> Sum3/3
  Gain/1 -> Sum2/3
  Ec_dq_n/1 -> Demux2/1
  Ic_dIq_n_Ref/1 -> Demux1/1
  Sum2/1 -> Mux/1
  Sum1/1 -> Divide3/1
  Divide2/1 -> PI Controller1/1
  Sum3/1 -> Mux/2
  Reset/1 -> PI Controller2/2, PI Controller1/2
  Constant3/1 -> Divide/2
  Constant/1 -> Divide/3
  Uc/1 -> Divide/4
  Constant6/1 -> Divide/5
  Divide1/1 -> Gain/1
  Divide4/1 -> Gain1/1
  Constant2/1 -> Divide1/2, Divide2/2, Divide4/2, Divide3/2
  Constant1/1 -> Divide3/3, Divide4/3, Divide1/3, Divide2/3
  PI Controller2/1 -> Sum3/2
  PI Controller1/1 -> Sum2/2

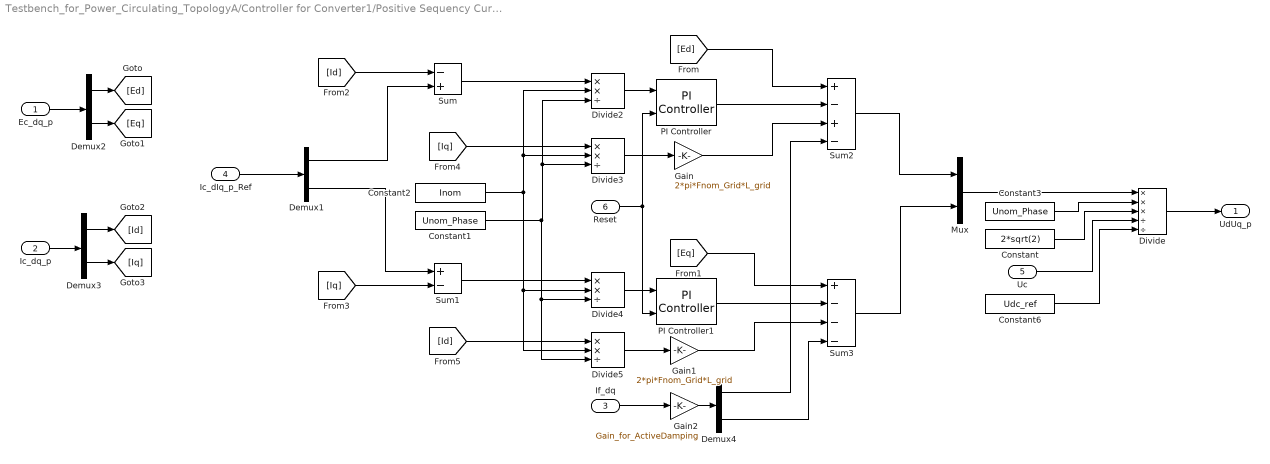
== system Testbench_for_Power_Circulating_TopologyA/Controller for Converter1/Positive Sequency Current Regulator ==
  Ec_dq_p : Inport
  Ic_dq_p : Inport  Port=2
  If_dq : Inport  Port=3
  Ic_dIq_p_Ref : Inport  Port=4
  Uc : Inport  Port=5
  Reset : Inport  Port=6  OutDataTypeStr=boolean
  Constant : Constant  Value=2*sqrt(2)  OutDataTypeStr=Inherit: Inherit via back propagation  SampleTime=-1
  Constant1 : Constant  Value=Unom_Phase  OutDataTypeStr=Inherit: Inherit via back propagation  SampleTime=-1
  Constant2 : Constant  Value=Inom  OutDataTypeStr=Inherit: Inherit via back propagation  SampleTime=-1
  Constant3 : Constant  Value=Unom_Phase  OutDataTypeStr=Inherit: Inherit via back propagation  SampleTime=-1
  Constant6 : Constant  Value=Udc_ref  OutDataTypeStr=Inherit: Inherit via back propagation  SampleTime=-1
  Demux{1..4} (4 alike) : Demux  Outputs=2
  Divide : Product  Inputs=***//  OutDataTypeStr=single
  Divide{2..5} (4 alike) : Product  Inputs=**/  OutDataTypeStr=single
  Gain : Gain  Gain=2*pi*Fnom_Grid*L_grid  ParamDataTypeStr=Inherit: Same as input
  Gain1 : Gain  Gain=2*pi*Fnom_Grid*L_grid  ParamDataTypeStr=Inherit: Same as input
  Gain2 : Gain  Gain=Gain_for_ActiveDamping  ParamDataTypeStr=Inherit: Same as input
  Mux : Mux  Inputs=2
  PI Controller : LibraryForCodeGeneration/PI Controller  Kp=Kp_Idq  Ki=Ki_Idq  Ts=Ts_Control  Max=2  Min=-2
  PI Controller1 : LibraryForCodeGeneration/PI Controller  Kp=Kp_Idq  Ki=Ki_Idq  Ts=Ts_Control  Max=2  Min=-2
  Sum : Sum  Inputs=-+  InputSameDT=on  SaturateOnIntegerOverflow=on  OutDataTypeStr=Inherit: Same as first input
  Sum1 : Sum  Inputs=+-  InputSameDT=on  SaturateOnIntegerOverflow=on  OutDataTypeStr=Inherit: Same as first input
  Sum2 : Sum  Inputs=+-+-  InputSameDT=on  SaturateOnIntegerOverflow=on  OutDataTypeStr=Inherit: Same as first input
  Sum3 : Sum  Inputs=+---  InputSameDT=on  SaturateOnIntegerOverflow=on  OutDataTypeStr=Inherit: Same as first input
  UdUq_p : Outport
  wires:
  Sum3/1 -> Mux/2
  Sum1/1 -> Divide4/1
  Sum2/1 -> Mux/1
  Ic_dIq_p_Ref/1 -> Demux1/1
  Uc/1 -> Divide/4
  Divide3/1 -> Gain/1
  Divide5/1 -> Gain1/1
  Ec_dq_p/1 -> Demux2/1
  Gain/1 -> Sum2/3
  Divide/1 -> UdUq_p/1
  Mux/1 -> Divide/1
  Sum/1 -> Divide2/1
  Divide4/1 -> PI Controller1/1
  Demux2/1 -> [Ed]
  Demux2/2 -> [Eq]
  [Ed] -> Sum2/1
  Demux1/1 -> Sum/2
  Demux1/2 -> Sum1/1
  Demux3/2 -> [Iq]
  Demux3/1 -> [Id]
  Ic_dq_p/1 -> Demux3/1
  [Id] -> Sum/1
  [Iq] -> Sum1/2
  [Iq] -> Divide3/1
  [Id] -> Divide5/1
  PI Controller/1 -> Sum2/2
  Divide2/1 -> PI Controller/1
  Reset/1 -> PI Controller1/2, PI Controller/2
  Constant3/1 -> Divide/2
  Constant/1 -> Divide/3
  Constant6/1 -> Divide/5
  Constant2/1 -> Divide5/2, Divide4/2, Divide3/2, Divide2/2
  Constant1/1 -> Divide5/3, Divide4/3, Divide3/3, Divide2/3
  If_dq/1 -> Gain2/1
  Demux4/1 -> Sum2/4
  Gain2/1 -> Demux4/1
  Demux4/2 -> Sum3/4
  [Eq] -> Sum3/1
  PI Controller1/1 -> Sum3/2
  Gain1/1 -> Sum3/3

== system Testbench_for_Power_Circulating_TopologyA/Controller for Converter1/Udq2Uabc ==
  Udq_p : Inport
  Udq_n : Inport  Port=2
  wt : Inport  Port=3
  Add : Sum
  Gain2 : Gain  Gain=-1  ParamDataTypeStr=Inherit: Same as input
  Saturation : Saturate  UpperLimit=1.15  LowerLimit=-1.15
  dq2abc : LibraryForCodeGeneration/dq2abc  SystemSampleTime=-1  VariantActivationTime=update diagram  AllowFlexibleInterface=on  Latency=0  AutoFrameSizeCalculation=off
  dq2abc1 : LibraryForCodeGeneration/dq2abc  SystemSampleTime=-1  VariantActivationTime=update diagram  AllowFlexibleInterface=on  Latency=0  AutoFrameSizeCalculation=off
  Uabc : Outport
  wires:
  dq2abc1/1 -> Add/2
  wt/1 -> dq2abc/2, Gain2/1
  Gain2/1 -> dq2abc1/2
  Udq_p/1 -> dq2abc/1
  Udq_n/1 -> dq2abc1/1
  Add/1 -> Saturation/1
  dq2abc/1 -> Add/1
  Saturation/1 -> Uabc/1

== system Testbench_for_Power_Circulating_TopologyA/Controller for Converter1/Voltage Regulator ==
  UDC : Inport
  Reset : Inport  Port=2
  Add : Sum  Inputs=+-
  Constant : Constant  Value=0  OutDataTypeStr=Inherit: Inherit via back propagation  SampleTime=-1
  Constant1 : Constant  OutDataTypeStr=single  SampleTime=-1
  Mux : Mux  Inputs=2
  Mux1 : Mux  Inputs=2
  PI Controller1 : LibraryForCodeGeneration/PI Controller  Kp=Kp_Udc  Ki=Ki_Udc  Ts=Ts_Control  Max=1.5  Min=-1.5
  Signal Conversion : SignalConversion  OverrideOpt=off
  Signal Conversion1 : SignalConversion  OverrideOpt=off
  IdIq_p_Ref : Outport
  IdIq_n_Ref : Outport  Port=2
  wires:
  Mux1/1 -> Signal Conversion1/1
  Mux/1 -> Signal Conversion/1
  UDC/1 -> Add/2
  PI Controller1/1 -> Mux/1
  Signal Conversion/1 -> IdIq_p_Ref/1  "Ic_dq_p_ref"
  Signal Conversion1/1 -> IdIq_n_Ref/1  "Ic_dq_n_ref"
  Constant/1 -> Mux1/1, Mux/2, Mux1/2
  Add/1 -> PI Controller1/1
  Reset/1 -> PI Controller1/2
  Constant1/1 -> Add/1

== system Testbench_for_Power_Circulating_TopologyA/Controller for Converter1/abc2dq_p1 ==
  "Ic_ABC_p " : Inport
  "Ic_ABC_n " : Inport  Port=2
  If_ABC : Inport  Port=3
  wt : Inport  Port=4
  Gain : Gain  Gain=-1
  abc2dq1 : LibraryForCodeGeneration/abc2dq  SystemSampleTime=-1  VariantActivationTime=update diagram  AllowFlexibleInterface=on  Latency=0  AutoFrameSizeCalculation=off
  abc2dq2 : LibraryForCodeGeneration/abc2dq  SystemSampleTime=-1  VariantActivationTime=update diagram  AllowFlexibleInterface=on  Latency=0  AutoFrameSizeCalculation=off
  abc2dq3 : LibraryForCodeGeneration/abc2dq  SystemSampleTime=-1  VariantActivationTime=update diagram  AllowFlexibleInterface=on  Latency=0  AutoFrameSizeCalculation=off
  Ic_dq_p : Outport
  If_dq : Outport  Port=2
  Ic_dq_n : Outport  Port=3
  wires:
  "Ic_ABC_p "/1 -> abc2dq1/1
  abc2dq1/1 -> Ic_dq_p/1
  If_ABC/1 -> abc2dq3/1
  abc2dq3/1 -> If_dq/1  "If_dq"
  Gain/1 -> abc2dq2/2  "Negetive_wt"
  "Ic_ABC_n "/1 -> abc2dq2/1
  abc2dq2/1 -> Ic_dq_n/1
  wt/1 -> abc2dq1/2, Gain/1, abc2dq3/2  "Ic_ABC_p"

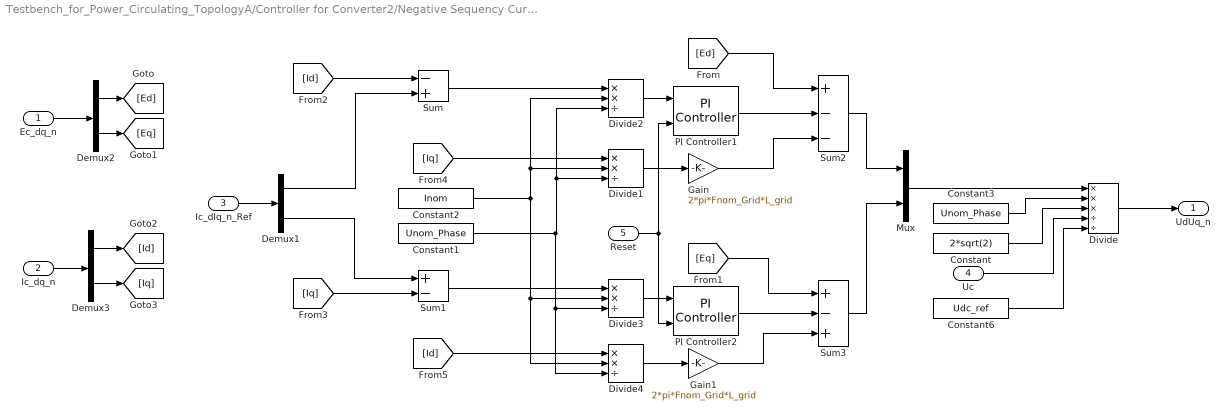
== system Testbench_for_Power_Circulating_TopologyA/Controller for Converter2/Negative Sequency Current Regulator ==
  Ec_dq_n : Inport
  Ic_dq_n : Inport  Port=2
  Ic_dIq_n_Ref : Inport  Port=3
  Uc : Inport  Port=4
  Reset : Inport  Port=5  OutDataTypeStr=boolean
  Constant : Constant  Value=2*sqrt(2)  OutDataTypeStr=Inherit: Inherit via back propagation  SampleTime=-1
  Constant1 : Constant  Value=Unom_Phase  OutDataTypeStr=Inherit: Inherit via back propagation  SampleTime=-1
  Constant2 : Constant  Value=Inom  OutDataTypeStr=Inherit: Inherit via back propagation  SampleTime=-1
  Constant3 : Constant  Value=Unom_Phase  OutDataTypeStr=Inherit: Inherit via back propagation  SampleTime=-1
  Constant6 : Constant  Value=Udc_ref  OutDataTypeStr=Inherit: Inherit via back propagation  SampleTime=-1
  Demux1 : Demux  Outputs=2
  Demux2 : Demux  Outputs=2
  Demux3 : Demux  Outputs=2
  Divide : Product  Inputs=***//  OutDataTypeStr=single
  Divide{1..4} (4 alike) : Product  Inputs=**/  OutDataTypeStr=single
  Gain : Gain  Gain=2*pi*Fnom_Grid*L_grid  ParamDataTypeStr=Inherit: Same as input
  Gain1 : Gain  Gain=2*pi*Fnom_Grid*L_grid  ParamDataTypeStr=Inherit: Same as input
  Mux : Mux  Inputs=2
  PI Controller1 : LibraryForCodeGeneration/PI Controller  Kp=Kp_Idq  Ki=Ki_Idq  Ts=Ts_Control  Max=2  Min=-2
  PI Controller2 : LibraryForCodeGeneration/PI Controller  Kp=Kp_Idq  Ki=Ki_Idq  Ts=Ts_Control  Max=2  Min=-2
  Sum : Sum  Inputs=-+  InputSameDT=on  SaturateOnIntegerOverflow=on  OutDataTypeStr=Inherit: Same as first input
  Sum1 : Sum  Inputs=+-  InputSameDT=on  SaturateOnIntegerOverflow=on  OutDataTypeStr=Inherit: Same as first input
  Sum2 : Sum  Inputs=+--  InputSameDT=on  SaturateOnIntegerOverflow=on  OutDataTypeStr=Inherit: Same as first input
  Sum3 : Sum  Inputs=+-+  InputSameDT=on  SaturateOnIntegerOverflow=on  OutDataTypeStr=Inherit: Same as first input
  UdUq_n : Outport
  wires:
  PI Controller1/1 -> Sum2/2
  PI Controller2/1 -> Sum3/2
  Constant1/1 -> Divide2/3, Divide1/3, Divide4/3, Divide3/3
  Constant2/1 -> Divide3/2, Divide4/2, Divide2/2, Divide1/2
  Divide4/1 -> Gain1/1
  Divide1/1 -> Gain/1
  Constant6/1 -> Divide/5
  Uc/1 -> Divide/4
  Constant/1 -> Divide/3
  Constant3/1 -> Divide/2
  Reset/1 -> PI Controller1/2, PI Controller2/2
  Sum3/1 -> Mux/2
  Divide2/1 -> PI Controller1/1
  Sum1/1 -> Divide3/1
  Sum2/1 -> Mux/1
  Ic_dIq_n_Ref/1 -> Demux1/1
  Ec_dq_n/1 -> Demux2/1
  Gain/1 -> Sum2/3
  Gain1/1 -> Sum3/3
  Divide/1 -> UdUq_n/1
  Mux/1 -> Divide/1
  Sum/1 -> Divide2/1
  Divide3/1 -> PI Controller2/1
  Demux2/1 -> [Ed]
  Demux2/2 -> [Eq]
  [Ed] -> Sum2/1
  [Eq] -> Sum3/1
  Demux1/1 -> Sum/2
  Demux1/2 -> Sum1/1
  Demux3/2 -> [Iq]
  Demux3/1 -> [Id]
  Ic_dq_n/1 -> Demux3/1
  [Id] -> Sum/1
  [Iq] -> Sum1/2
  [Iq] -> Divide1/1
  [Id] -> Divide4/1

== system Testbench_for_Power_Circulating_TopologyA/Controller for Converter2/PQ2Idq ==
  PQ_Ref : Inport
  Constant : Constant  Value=0  OutDataTypeStr=Inherit: Inherit via back propagation  SampleTime=-1
  Demux : Demux  Outputs=2
  Mux : Mux  Inputs=2
  Mux1 : Mux  Inputs=2
  Signal Conversion : SignalConversion  OverrideOpt=off
  Signal Conversion1 : SignalConversion  OverrideOpt=off
  IdIq_p_Ref : Outport
  IdIq_n_Ref : Outport  Port=2
  wires:
  Constant/1 -> Mux1/1, Mux1/2
  Signal Conversion1/1 -> IdIq_n_Ref/1  "Ic_dq_n_ref"
  Signal Conversion/1 -> IdIq_p_Ref/1  "Ic_dq_p_ref"
  Demux/1 -> Mux/1
  Demux/2 -> Mux/2
  PQ_Ref/1 -> Demux/1  "PQ_REF"
  Mux/1 -> Signal Conversion/1
  Mux1/1 -> Signal Conversion1/1

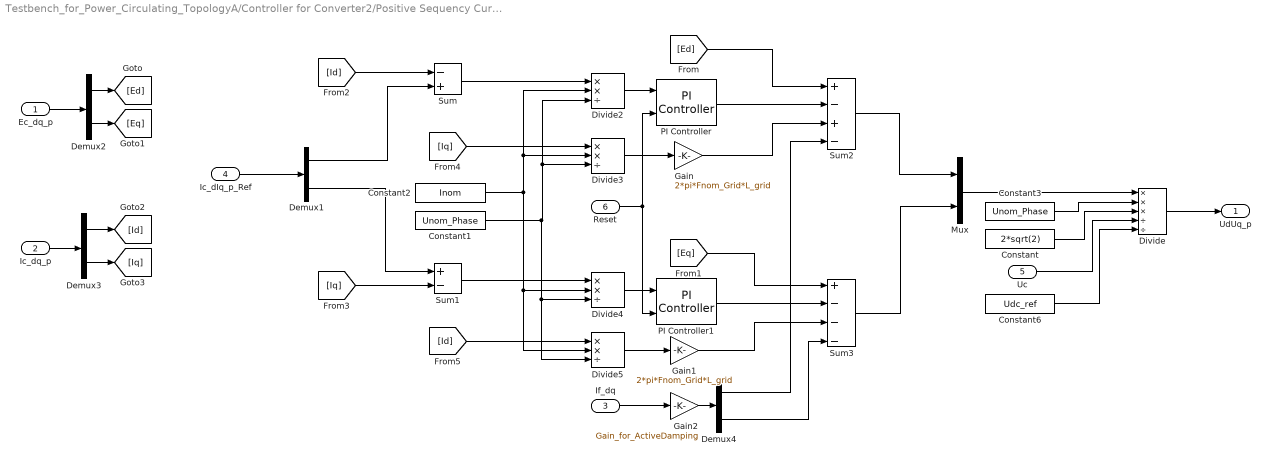
== system Testbench_for_Power_Circulating_TopologyA/Controller for Converter2/Positive Sequency Current Regulator ==
  Ec_dq_p : Inport
  Ic_dq_p : Inport  Port=2
  If_dq : Inport  Port=3
  Ic_dIq_p_Ref : Inport  Port=4
  Uc : Inport  Port=5
  Reset : Inport  Port=6  OutDataTypeStr=boolean
  Constant : Constant  Value=2*sqrt(2)  OutDataTypeStr=Inherit: Inherit via back propagation  SampleTime=-1
  Constant1 : Constant  Value=Unom_Phase  OutDataTypeStr=Inherit: Inherit via back propagation  SampleTime=-1
  Constant2 : Constant  Value=Inom  OutDataTypeStr=Inherit: Inherit via back propagation  SampleTime=-1
  Constant3 : Constant  Value=Unom_Phase  OutDataTypeStr=Inherit: Inherit via back propagation  SampleTime=-1
  Constant6 : Constant  Value=Udc_ref  OutDataTypeStr=Inherit: Inherit via back propagation  SampleTime=-1
  Demux{1..4} (4 alike) : Demux  Outputs=2
  Divide : Product  Inputs=***//  OutDataTypeStr=single
  Divide{2..5} (4 alike) : Product  Inputs=**/  OutDataTypeStr=single
  Gain : Gain  Gain=2*pi*Fnom_Grid*L_grid  ParamDataTypeStr=Inherit: Same as input
  Gain1 : Gain  Gain=2*pi*Fnom_Grid*L_grid  ParamDataTypeStr=Inherit: Same as input
  Gain2 : Gain  Gain=Gain_for_ActiveDamping  ParamDataTypeStr=Inherit: Same as input
  Mux : Mux  Inputs=2
  PI Controller : LibraryForCodeGeneration/PI Controller  Kp=Kp_Idq  Ki=Ki_Idq  Ts=Ts_Control  Max=2  Min=-2
  PI Controller1 : LibraryForCodeGeneration/PI Controller  Kp=Kp_Idq  Ki=Ki_Idq  Ts=Ts_Control  Max=2  Min=-2
  Sum : Sum  Inputs=-+  InputSameDT=on  SaturateOnIntegerOverflow=on  OutDataTypeStr=Inherit: Same as first input
  Sum1 : Sum  Inputs=+-  InputSameDT=on  SaturateOnIntegerOverflow=on  OutDataTypeStr=Inherit: Same as first input
  Sum2 : Sum  Inputs=+-+-  InputSameDT=on  SaturateOnIntegerOverflow=on  OutDataTypeStr=Inherit: Same as first input
  Sum3 : Sum  Inputs=+---  InputSameDT=on  SaturateOnIntegerOverflow=on  OutDataTypeStr=Inherit: Same as first input
  UdUq_p : Outport
  wires:
  Gain1/1 -> Sum3/3
  PI Controller1/1 -> Sum3/2
  [Eq] -> Sum3/1
  Demux4/2 -> Sum3/4
  Gain2/1 -> Demux4/1
  Demux4/1 -> Sum2/4
  If_dq/1 -> Gain2/1
  Constant1/1 -> Divide2/3, Divide3/3, Divide4/3, Divide5/3
  Constant2/1 -> Divide2/2, Divide3/2, Divide4/2, Divide5/2
  Constant6/1 -> Divide/5
  Constant/1 -> Divide/3
  Constant3/1 -> Divide/2
  Reset/1 -> PI Controller/2, PI Controller1/2
  Divide2/1 -> PI Controller/1
  PI Controller/1 -> Sum2/2
  [Id] -> Divide5/1
  [Iq] -> Divide3/1
  [Iq] -> Sum1/2
  [Id] -> Sum/1
  Ic_dq_p/1 -> Demux3/1
  Demux3/1 -> [Id]
  Demux3/2 -> [Iq]
  Demux1/2 -> Sum1/1
  Demux1/1 -> Sum/2
  [Ed] -> Sum2/1
  Demux2/2 -> [Eq]
  Demux2/1 -> [Ed]
  Divide4/1 -> PI Controller1/1
  Sum/1 -> Divide2/1
  Mux/1 -> Divide/1
  Divide/1 -> UdUq_p/1
  Gain/1 -> Sum2/3
  Ec_dq_p/1 -> Demux2/1
  Divide5/1 -> Gain1/1
  Divide3/1 -> Gain/1
  Uc/1 -> Divide/4
  Ic_dIq_p_Ref/1 -> Demux1/1
  Sum2/1 -> Mux/1
  Sum1/1 -> Divide4/1
  Sum3/1 -> Mux/2

== system Testbench_for_Power_Circulating_TopologyA/Controller for Converter2/Udq2Uabc ==
  Udq_p : Inport
  Udq_n : Inport  Port=2
  wt : Inport  Port=3
  Add : Sum
  Gain2 : Gain  Gain=-1  ParamDataTypeStr=Inherit: Same as input
  Saturation : Saturate  UpperLimit=1.15  LowerLimit=-1.15
  dq2abc : LibraryForCodeGeneration/dq2abc  SystemSampleTime=-1  VariantActivationTime=update diagram  AllowFlexibleInterface=on  Latency=0  AutoFrameSizeCalculation=off
  dq2abc1 : LibraryForCodeGeneration/dq2abc  SystemSampleTime=-1  VariantActivationTime=update diagram  AllowFlexibleInterface=on  Latency=0  AutoFrameSizeCalculation=off
  Uabc : Outport
  wires:
  Saturation/1 -> Uabc/1
  dq2abc/1 -> Add/1
  Add/1 -> Saturation/1
  Udq_n/1 -> dq2abc1/1
  Udq_p/1 -> dq2abc/1
  Gain2/1 -> dq2abc1/2
  wt/1 -> Gain2/1, dq2abc/2
  dq2abc1/1 -> Add/2

== system Testbench_for_Power_Circulating_TopologyA/Controller for Converter2/abc2dq_p1 ==
  "Ic_ABC_p " : Inport
  "Ic_ABC_n " : Inport  Port=2
  If_ABC : Inport  Port=3
  wt : Inport  Port=4
  Gain : Gain  Gain=-1
  abc2dq1 : LibraryForCodeGeneration/abc2dq  SystemSampleTime=-1  VariantActivationTime=update diagram  AllowFlexibleInterface=on  Latency=0  AutoFrameSizeCalculation=off
  abc2dq2 : LibraryForCodeGeneration/abc2dq  SystemSampleTime=-1  VariantActivationTime=update diagram  AllowFlexibleInterface=on  Latency=0  AutoFrameSizeCalculation=off
  abc2dq3 : LibraryForCodeGeneration/abc2dq  SystemSampleTime=-1  VariantActivationTime=update diagram  AllowFlexibleInterface=on  Latency=0  AutoFrameSizeCalculation=off
  Ic_dq_p : Outport
  If_dq : Outport  Port=2
  Ic_dq_n : Outport  Port=3
  wires:
  wt/1 -> abc2dq3/2, Gain/1, abc2dq1/2  "Ic_ABC_p"
  abc2dq2/1 -> Ic_dq_n/1
  "Ic_ABC_n "/1 -> abc2dq2/1
  Gain/1 -> abc2dq2/2  "Negetive_wt"
  abc2dq3/1 -> If_dq/1  "If_dq"
  If_ABC/1 -> abc2dq3/1
  abc2dq1/1 -> Ic_dq_p/1
  "Ic_ABC_p "/1 -> abc2dq1/1

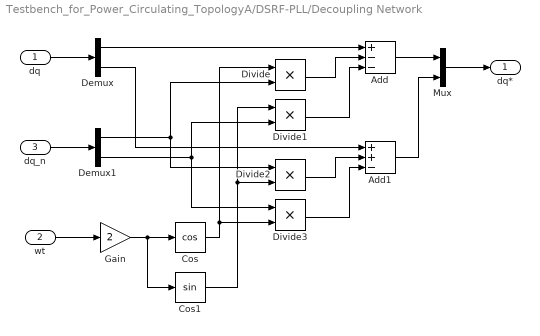
== system Testbench_for_Power_Circulating_TopologyA/DSRF-PLL/Decoupling Network ==
  dq : Inport
  wt : Inport  Port=2
  dq_n : Inport  Port=3
  Add : Sum  Inputs=+--  OutDataTypeStr=Inherit: Same as first input
  Add1 : Sum  Inputs=++-  OutDataTypeStr=Inherit: Same as first input
  Cos : Trigonometry  Operator=cos
  Cos1 : Trigonometry
  Demux : Demux  Outputs=2
  Demux1 : Demux  Outputs=2
  Divide{,1..3} (4 alike) : Product  Inputs=**
  Gain : Gain  Gain=2
  Mux : Mux  Inputs=2
  dq* : Outport
  wires:
  Add1/1 -> Mux/2
  Demux/2 -> Add1/1
  Divide3/1 -> Add1/3
  Divide2/1 -> Add1/2
  Mux/1 -> dq*/1
  Add/1 -> Mux/1
  Divide1/1 -> Add/3
  Demux1/2 -> Divide1/2, Divide3/1
  Cos1/1 -> Divide1/1, Divide2/2
  Demux1/1 -> Divide/2, Divide2/1
  dq_n/1 -> Demux1/1
  Cos/1 -> Divide/1, Divide3/2
  Divide/1 -> Add/2
  Demux/1 -> Add/1
  Gain/1 -> Cos/1, Cos1/1
  dq/1 -> Demux/1
  wt/1 -> Gain/1

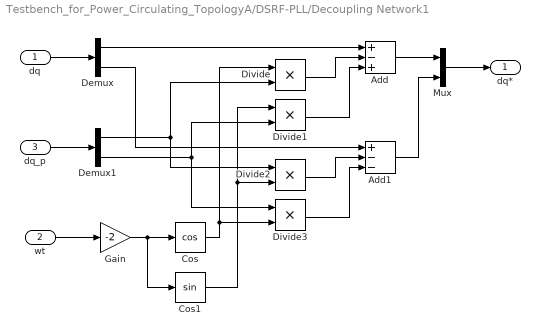
== system Testbench_for_Power_Circulating_TopologyA/DSRF-PLL/Decoupling Network1 ==
  dq : Inport
  wt : Inport  Port=2
  dq_p : Inport  Port=3
  Add : Sum  Inputs=+-+  OutDataTypeStr=Inherit: Same as first input
  Add1 : Sum  Inputs=+--  OutDataTypeStr=Inherit: Same as first input
  Cos : Trigonometry  Operator=cos
  Cos1 : Trigonometry
  Demux : Demux  Outputs=2
  Demux1 : Demux  Outputs=2
  Divide{,1..3} (4 alike) : Product  Inputs=**
  Gain : Gain  Gain=-2
  Mux : Mux  Inputs=2
  dq* : Outport
  wires:
  Mux/1 -> dq*/1
  Gain/1 -> Cos/1, Cos1/1
  Demux/1 -> Add/1
  Cos1/1 -> Divide1/1, Divide2/2
  dq/1 -> Demux/1
  Demux1/2 -> Divide1/2, Divide3/1
  Cos/1 -> Divide/1, Divide3/2
  Demux1/1 -> Divide/2, Divide2/1
  dq_p/1 -> Demux1/1
  Divide1/1 -> Add/3
  Add1/1 -> Mux/2
  Add/1 -> Mux/1
  Divide2/1 -> Add1/2
  Divide3/1 -> Add1/3
  Demux/2 -> Add1/1
  wt/1 -> Gain/1
  Divide/1 -> Add/2

== system Testbench_for_Power_Circulating_TopologyA/DSRF-PLL/Discreted First Order Low-Pass Filter ==
  u : Inport
  Add3 : Sum  Inputs=|+-
  Delay : Delay  DelayLength=1
  Gain1 : Gain  Gain=Ts*Wc-1
  Gain2 : Gain  Gain=Ts*Wc
  y : Outport
  wires:
  Gain2/1 -> y/1
  Delay/1 -> Gain1/1, Gain2/1
  Gain1/1 -> Add3/2
  u/1 -> Add3/1
  Add3/1 -> Delay/1
